simulink model "Final_Model_Building_2_AirflowAdded"  (R2022a)
settings: Solver=ode1  StartTime=0.0  StopTime=24*3600  FixedStep=10  RelTol=1e-3
values from neighbouring files (symbols this model uses):
  Aux_Threshold = 52    [Setup_Code_EWASP_VC.m]
  buildingAge = 2005    [Setup_Code_EWASP_VC.m]
  ceilingHeight = 2.4    [Setup_Code_EWASP_VC.m]
  conductiveHconnectMatrix = [ ... (first row only)    [Setup_Code_EWASP_VC.m]
  cRoofGreen = 100000    [Setup_Code_EWASP_VC.m]
  Defrost_After_Time = 30    [Setup_Code_EWASP_VC.m]
  DHWDemandProfile = occFreegainHotwaterElecTestPassiveOcc3(:,3)    [Setup_Code_EWASP_VC.m]
  Elec_Max = Elec_Max*(30/24.2)    [Setup_Code_EWASP_VC.m]
  Elec_Mid = Elec_Mid*(30/24.2)    [Setup_Code_EWASP_VC.m]
  Elec_Min = Elec_Min*(30/24.2)    [Setup_Code_EWASP_VC.m]
  ElecDemandProfile = occFreegainHotwaterElecTestPassiveOcc3(:,4)    [Setup_Code_EWASP_VC.m]
  ElecFixed = [Elec_Max(6,2) Elec_Max(6,4) Elec_Max(6,6) Elec_Max(6,7) ... (first row only)    [Setup_Code_EWASP_VC.m]
  floorOrCeilingArea = floorOrCeilingArea*1.15    [Setup_Code_EWASP_VC.m]
  forceCold = 0    [Setup_Code_EWASP_VC.m]
  freegain = occFreegainHotwaterElecTestPassiveOcc3(:,2)-max(occupancy)*25    [Setup_Code_EWASP_VC.m]
  furnitureModelOn = 1    [Setup_Code_EWASP_VC.m]
  Heat_Max = Heat_Max*(30/24.2)    [Setup_Code_EWASP_VC.m]
  Heat_Mid = Heat_Mid*(30/24.2)    [Setup_Code_EWASP_VC.m]
  Heat_Min = Heat_Min*(30/24.2)    [Setup_Code_EWASP_VC.m]
  HeatFixed = [Heat_Max(6,2) Heat_Max(6,4) Heat_Max(6,6) Heat_Max(6,7) ... (first row only)    [Setup_Code_EWASP_VC.m]
  HeatingOnProfile = repmat(HeatingOnProfile,365,1)    [Setup_Code_EWASP_VC.m]
  HEX_ReturnLowerLimit = 52.5    [Setup_Code_EWASP_VC.m]
  HEX_ReturnUpperLimit = 55    [Setup_Code_EWASP_VC.m]
  LeakMultiplier = 1+(2*(rand()-0.5)/10)    [Setup_Code_EWASP_VC.m]
  maxOcc = max(occupancyProfile)    [Setup_Code_EWASP_VC.m]
  NESW_wallArea = max(NESW_Lengths*ceilingHeight-NESW_Windows,0)    [Setup_Code_EWASP_VC.m]
  NESW_Windows = [ ... (first row only)    [Setup_Code_EWASP_VC.m]
  numRooms = roomCount    [Setup_Code_EWASP_VC.m]
  occupancy = occupancyProfile    [Setup_Code_EWASP_VC.m]
  offsetDays = 0    [Setup_Code_EWASP_VC.m]
  pumpChoice = pumpChoices(MinIndex,1)    [Setup_Code_EWASP_VC.m]
  pumpRamp = 180    [Setup_Code_EWASP_VC.m]
  ReturnLowerLimit = 37.5    [Setup_Code_EWASP_VC.m]
  ReturnUpperLimit = 40    [Setup_Code_EWASP_VC.m]
  RoofIrradiance = Flat_NS_EW_RoofIrradiance(:,1)    [Setup_Code_EWASP_VC.m]
  roofStartTemp = ones(11,1)*20    [Setup_Code_EWASP_VC.m]
  rooftype = 0    [Setup_Code_EWASP_VC.m]
  RoomDataMatrix = [zeros(1,12);ones(1,12)*wallDensity;zeros(1,12);ones(1,12)*wallU;ones(1,12)*windowU;ones(1,12)*floorU;ones(1,12)*ceilingU;zeros(1,12);windowArea, 0;floorOrCeilingArea;zeros(1,12);floorOrCeilingArea*ceilingHeight]    [Setup_Code_EWASP_VC.m]
  roomVol = roomVol*1.15    [Setup_Code_EWASP_VC.m]
  slabStartTemp = (GroundTempTimeSeries(offsetDays*1440+1,1)+thermostatSetting)/2    [Setup_Code_EWASP_VC.m]
  SlackRequest = zeros(1440,1)    [Setup_Code_EWASP_VC.m]
  SolarThermalExists = 0    [Setup_Code_EWASP_VC.m]
  SourceFixed = HeatFixed-ElecFixed    [Setup_Code_EWASP_VC.m]
  StateSeries = StateSeriesGenerator(22,7,1)    [Setup_Code_EWASP_VC.m]
  Tank_Lower_Temp = 49.5    [Setup_Code_EWASP_VC.m]
  Tank_Upper_Temp = 52    [Setup_Code_EWASP_VC.m]
  Tank_Volume_m3 = 0.15    [Setup_Code_EWASP_VC.m]
  TankHeatHour = randi([1 5])-1    [Setup_Code_EWASP_VC.m]
  upDown = [0;0;0;0;1;1;1;1;1;1;1]    [Setup_Code_EWASP_VC.m]
  wallStartTempExt = thermostatSetting*(0.266+0.00215*outdoorStartTemp+0.018*wallU+0.00113*outdoorStartTemp*wallU+0.0068*wallU^2)    [Setup_Code_EWASP_VC.m]
undefined symbols (not defined in the file or in its folder): a, ceilingU, condUDMatrix, convUDMatrix, deltaPEXPANDED_E, deltaPEXPANDED_E2, deltaPEXPANDED_N, deltaPEXPANDED_N2, deltaPEXPANDED_S, deltaPEXPANDED_S2, deltaPEXPANDED_W, deltaPEXPANDED_W2, DesiredDHWTemp, DesiredFlowTempVsInOutDeltaTemp, DiffuseHorizontal, DiscIntNeverNeededParam, DNI, dwnAndConcrete, DWORK_A_HX, DWORK_CHK_FLU, DWORK_CP_NODE, DWORK_DH, DWORK_FLUID, DWORK_HCON, DWORK_LOSS, DWORK_MDOTDOWN, DWORK_MDOTIN, DWORK_MDOTUP, DWORK_MIX, DWORK_PRESS, DWORK_QDOTIN, DWORK_RHO_NODE, DWORK_TIN, DWORK_TS_OLD, DWORK_V_NODE, ExtractRates, GroundTempTimeSeries, HCM, HCM2, HCM_closed, HCM_closed2, intermediateU, IsTop, massFlowMatrix, mechEfficiency, neighbourMatrix, numericalRoomUse, RadiatorMatrix, room2roomflowmatrix_E, room2roomflowmatrix_E2, room2roomflowmatrix_N, room2roomflowmatrix_N2, room2roomflowmatrix_S, room2roomflowmatrix_S2, room2roomflowmatrix_W, room2roomflowmatrix_W2, StateAirInEXPANDED_E, StateAirInEXPANDED_E2, StateAirInEXPANDED_N, StateAirInEXPANDED_N2 ... (+27)
libraries: simulink x6, dspsigops x4, dspmtrx3 x4, carnot x3, spsEdgeDetectorLib x2, dspstat3 x2, powerlib_meascontrol x1, simulink_extras x1
(part 16 of 27)

== system Final_Model_Building_2_AirflowAdded/Subsystem_Room3/Utility/Subsystem7 ==
  note: Q from room to ground
  In1 : Inport
  In2 : Inport  Port=2
  In3 : Inport  Port=3
  In4 : Inport  Port=4
  In5 : Inport  Port=5
  In6 : Inport  Port=6
  In7 : Inport  Port=7
  In8 : Inport  Port=8
  C per kg : Constant  Value=1000
  C per kg1 : Constant  Value=0.25
  Density : Constant  Value=2350
  Floor heat capacity total : Product  Inputs=4
  Product : Product  Inputs=3
  Product1 : Product  Inputs=3
  Product2 : Product  Inputs=*/
  QlossFromNodetoGround : Product  Inputs=3
  Sum : Sum  Inputs=+-
  Sum1 : Sum  Inputs=+-
  Sum2 : Sum
  Tchange node to ground : Product  Inputs=*/
  Thickness : Constant  Value=0.2
  deltaTNode-Ground : Sum  Inputs=+-
  doubler : Constant  Value=2
  halfUVal : Product
  "house has green roof, and the room is on the top floor" : Constant
  subtract room-concret loss from conrete-earth loss : Sum  Inputs=-+
  "switches off normal house roof loss if a green or passive roof is selected, and the room is on the top floor" : Switch  Criteria=u2 > Threshold  Threshold=0.5  SaturateOnIntegerOverflow=off  InputSameDT=off
  z : Constant  Value=0
  Out1 : Outport  VectorParamsAs1DForOutWhenUnconnected=off
  Out2 : Outport  Port=2  VectorParamsAs1DForOutWhenUnconnected=off
  wires:
  In6/1 -> Product1/3
  Sum/1 -> Product/1
  In1/1 -> Sum/1, Sum1/1
  In2/1 -> deltaTNode-Ground/2
  In4/1 -> Floor heat capacity total/1, Product1/2, Product/2, QlossFromNodetoGround/2
  Sum1/1 -> Product1/1
  "switches off normal house roof loss if a green or passive roof is selected, and the room is on the top floor"/1 -> Sum2/2
  In5/1 -> halfUVal/2
  In3/1 -> Sum1/2
  Sum2/1 -> Product2/1
  In7/1 -> Product2/2
  Product2/1 -> Out1/1
  C per kg/1 -> Floor heat capacity total/2
  Density/1 -> Floor heat capacity total/4
  Thickness/1 -> Floor heat capacity total/3
  In8/1 -> Sum/2, deltaTNode-Ground/1
  doubler/1 -> halfUVal/1
  deltaTNode-Ground/1 -> QlossFromNodetoGround/1
  halfUVal/1 -> QlossFromNodetoGround/3
  Floor heat capacity total/1 -> Tchange node to ground/2
  Product/1 -> subtract room-concret loss from conrete-earth loss/1, Sum2/1
  QlossFromNodetoGround/1 -> subtract room-concret loss from conrete-earth loss/2
  subtract room-concret loss from conrete-earth loss/1 -> Tchange node to ground/1
  Tchange node to ground/1 -> Out2/1
  C per kg1/1 -> Product/3
  Product1/1 -> "switches off normal house roof loss if a green or passive roof is selected, and the room is on the top floor"/3
  z/1 -> "switches off normal house roof loss if a green or passive roof is selected, and the room is on the top floor"/1
  "house has green roof, and the room is on the top floor"/1 -> "switches off normal house roof loss if a green or passive roof is selected, and the room is on the top floor"/2

== system Final_Model_Building_2_AirflowAdded/Subsystem_Room3/Utility/furniture ==
  In1 : Inport
  In2 : Inport  Port=2
  In3 : Inport  Port=3
  Constant3 : Constant  Value=20
  Constant4 : Constant  Value=20
  Discrete-Time Integrator : DiscreteIntegrator  InitialConditionSource=external  SampleTime=-1  ICPrevOutput=DiscIntNeverNeededParam  ICPrevScaledInput=DiscIntNeverNeededParam
  Discrete-Time Integrator1 : DiscreteIntegrator  InitialConditionSource=external  SampleTime=-1  ICPrevOutput=DiscIntNeverNeededParam  ICPrevScaledInput=DiscIntNeverNeededParam
  MATLAB Function : MATLAB Function  TreatAsAtomicUnit=on
  Plus1 : Sum
  Out1 : Outport  VectorParamsAs1DForOutWhenUnconnected=off
  wires:
  [A1] -> Discrete-Time Integrator/1
  Constant4/1 -> Discrete-Time Integrator1/2
  [B1] -> Discrete-Time Integrator1/1
  Constant3/1 -> Discrete-Time Integrator/2
  Discrete-Time Integrator/1 -> MATLAB Function/4(TemperatureWoodPlastic)
  Discrete-Time Integrator1/1 -> MATLAB Function/5(TemperatureSoft)
  MATLAB Function/2(deltaTWoodPlasticMean) -> [A1]
  MATLAB Function/4(deltaTsoftMean) -> [B1]
  MATLAB Function/3(softHeatTransfertoroom) -> Plus1/2
  MATLAB Function/1(woodPlasticHeatTransfertoroom) -> Plus1/1
  In3/1 -> MATLAB Function/3(roomTemp)
  In1/1 -> MATLAB Function/1(roomArea)
  Plus1/1 -> Out1/1
  In2/1 -> MATLAB Function/2(roomtype)

== system Final_Model_Building_2_AirflowAdded/Subsystem_Room4/Hall/Radiator w//Thermostatic Control1 ==
  In1 : Inport
  In3 : Inport  Port=2
  In2 : Inport  Port=3
  Add : Sum  Inputs=+-
  Constant : Constant  Value=Water_Volume
  Constant1 : Constant  Value=TRV_Therm_Setpoint
  Constant11 : Constant  Value=0
  Constant2 : Constant  Value=0.5
  Constant3 : Constant  Value=4180
  Constant6 : Constant  Value=40
  Constant7 : Constant  Value=40
  Discrete-Time Integrator : DiscreteIntegrator  InitialConditionSource=external  SampleTime=-1  ICPrevOutput=DiscIntNeverNeededParam  ICPrevScaledInput=DiscIntNeverNeededParam
  Discrete-Time Integrator1 : DiscreteIntegrator  InitialConditionSource=external  SampleTime=-1  ICPrevOutput=DiscIntNeverNeededParam  ICPrevScaledInput=DiscIntNeverNeededParam
  From : From
  Goto : Goto
  MATLAB Function : MATLAB Function  TreatAsAtomicUnit=on
  Product2 : Product
  Qdot2room1 : Scope
  Real-Imag to Complex : RealImagToComplex
  Saturation : Saturate  UpperLimit=1  LowerLimit=0
  Scope1 : Scope
  Sum2 : Sum
  const1 : Constant  Value=Power_Nominal
  dTnom : Constant  Value=DeltaT_Nominal
  Out3 : Outport  VectorParamsAs1DForOutWhenUnconnected=off
  Out1 : Outport  Port=2  VectorParamsAs1DForOutWhenUnconnected=off
  Out2 : Outport  Port=3  VectorParamsAs1DForOutWhenUnconnected=off
  wires:
  In1/1 -> MATLAB Function/9(Troom), Add/2
  In2/1 -> Product2/1
  Constant1/1 -> Add/1
  Add/1 -> Sum2/1
  Constant2/1 -> Sum2/2
  Sum2/1 -> Saturation/1
  Saturation/1 -> Qdot2room1/1, Product2/2
  Constant11/1 -> Real-Imag to Complex/2
  Discrete-Time Integrator/1 -> MATLAB Function/5(Tnode1)
  Real-Imag to Complex/1 -> MATLAB Function/8(nominalDeltaT)
  MATLAB Function/3(Qtoroom) -> Out3/1, Scope1/1
  Product2/1 -> MATLAB Function/3(mdotRad), Out2/1
  Constant3/1 -> MATLAB Function/2(heatCapRad)
  const1/1 -> MATLAB Function/7(nominalHeat)
  [B] -> Discrete-Time Integrator1/1
  Constant6/1 -> Discrete-Time Integrator/2
  dTnom/1 -> Real-Imag to Complex/1
  Constant7/1 -> Discrete-Time Integrator1/2
  MATLAB Function/1(deltaT1) -> Goto/1
  MATLAB Function/2(deltaT2) -> [B]
  Discrete-Time Integrator1/1 -> Out1/1, MATLAB Function/6(Tnode2)
  Constant/1 -> MATLAB Function/1(MassRad)
  In3/1 -> MATLAB Function/4(Tflow)
  From/1 -> Discrete-Time Integrator/1

== system Final_Model_Building_2_AirflowAdded/Subsystem_Room4/Hall/Subsystem1 ==
  In1 : Inport
  In2 : Inport  Port=2
  In3 : Inport  Port=3
  In4 : Inport  Port=4
  In5 : Inport  Port=5
  Add : Sum
  Constant1 : Constant  Value=TemperatureSeries
  Constant2 : Constant  Value=offsetDays
  Constant3 : Constant  Value=0.3
  Constant4 : Constant  Value=offsetDays
  Digital Clock : DigitalClock  SampleTime=10
  Digital Clock1 : DigitalClock  SampleTime=10
  MATLAB Function : MATLAB Function  TreatAsAtomicUnit=on
  MATLAB Function1 : MATLAB Function  TreatAsAtomicUnit=on
  RoomNodeNumber1 : Constant  Value=wallHeatCapacityInt
  RoomNodeNumber2 : Constant  Value=Wall_Irradiance_Angles_NEWS
  RoomNodeNumber3 : Constant  Value=DNI
  RoomNodeNumber4 : Constant  Value=DiffuseHorizontal
  RoomNodeNumber5 : Constant  Value=NESW_wallArea
  RoomNodeNumber6 : Constant  Value=NESW_wallArea
  RoomNodeNumber7 : Constant  Value=wallHeatCapacityMid
  RoomNodeNumber8 : Constant  Value=wallHeatCapacityExt
  Scope : Scope
  Scope1 : Scope
  Scope2 : Scope  NumInputPorts=3
  Scope3 : Scope
  Terminator : Terminator
  Terminator1 : Terminator
  Windspeed : Constant  Value=windSpeedSeries
  integrate deltat's with initial wall temps as initial condition : Subsystem
  sum to give HEAT LOST (i.e. positive value is a loss) : Sum  Inputs=+
  uVal_Total for wall : Constant  Value=wallU
  Out1 : Outport  VectorParamsAs1DForOutWhenUnconnected=off
  Out2 : Outport  Port=2  VectorParamsAs1DForOutWhenUnconnected=off
  Out3 : Outport  Port=3  VectorParamsAs1DForOutWhenUnconnected=off
  Out4 : Outport  Port=4  VectorParamsAs1DForOutWhenUnconnected=off
  wires:
  Constant1/1 -> MATLAB Function/9(T_AmbientSeries)
  integrate deltat's with initial wall temps as initial condition/1(Out1) -> Scope2/1, MATLAB Function/5(T_InWallNEWS)
  RoomNodeNumber2/1 -> MATLAB Function1/1(angleSeries)
  RoomNodeNumber1/1 -> MATLAB Function/2(c_InPU)
  MATLAB Function/2(deltaTmid) -> Out3/1
  In5/1 -> MATLAB Function/8(T_Room)
  MATLAB Function1/2(NEWS_Irradiance) -> Terminator1/1
  MATLAB Function/4(logRoomHeatLoss) -> sum to give HEAT LOST (i.e. positive value is a loss)/1, Scope/1
  RoomNodeNumber8/1 -> MATLAB Function/4(c_OutPU), MATLAB Function1/9(c_OutPU)
  uVal_Total for wall/1 -> MATLAB Function/1(uValWall)
  In4/1 -> integrate deltat's with initial wall temps as initial condition/3(In3)
  Digital Clock/1 -> MATLAB Function1/4(Time)
  integrate deltat's with initial wall temps as initial condition/2(Out2) -> Scope2/2, Scope1/1, MATLAB Function/6(T_MidWallNEWS)
  RoomNodeNumber7/1 -> MATLAB Function/3(c_MidPU)
  RoomNodeNumber3/1 -> MATLAB Function1/2(DNISeries)
  integrate deltat's with initial wall temps as initial condition/3(Out3) -> Scope2/3, MATLAB Function/7(T_OutWallNEWS)
  MATLAB Function/1(deltaTint) -> Out2/1
  MATLAB Function/3(deltaTout) -> Add/2
  In3/1 -> integrate deltat's with initial wall temps as initial condition/2(In2)
  Windspeed/1 -> MATLAB Function/10(windSpeedSeries)
  Constant3/1 -> MATLAB Function1/6(SurfaceAlbedo)
  RoomNodeNumber4/1 -> MATLAB Function1/3(DiffSeries)
  In1/1 -> integrate deltat's with initial wall temps as initial condition/4(In4), Scope3/1, MATLAB Function/12(roomNumber), MATLAB Function1/8(roomNumber)
  MATLAB Function1/3(deltaTexternalNEWS) -> Add/1
  RoomNodeNumber5/1 -> MATLAB Function1/7(NESW_wallArea)
  RoomNodeNumber6/1 -> MATLAB Function/11(NESW_wallArea)
  Constant4/1 -> MATLAB Function/14(offsetDays)
  Constant2/1 -> MATLAB Function1/5(offsetDays)
  Digital Clock1/1 -> MATLAB Function/13(Time)
  MATLAB Function1/1(PU_AreaIrradianceTotal) -> Terminator/1
  In2/1 -> integrate deltat's with initial wall temps as initial condition/1(In1)
  sum to give HEAT LOST (i.e. positive value is a loss)/1 -> Out4/1
  Add/1 -> Out1/1

== system Final_Model_Building_2_AirflowAdded/Subsystem_Room4/Hall/Subsystem2 ==
  In1 : Inport
  In2 : Inport  Port=2
  Constant9 : Constant  Value=-1
  Direct Lookup Table (n-D) : LookupNDDirect  NumberOfTableDimensions=1  TableIsInput=on
  Plus : Sum
  Out1 : Outport  VectorParamsAs1DForOutWhenUnconnected=off
  wires:
  Plus/1 -> Direct Lookup Table (n-D)/1
  Direct Lookup Table (n-D)/1 -> Out1/1
  Constant9/1 -> Plus/2
  In1/1 -> Plus/1
  In2/1 -> Direct Lookup Table (n-D)/2

== system Final_Model_Building_2_AirflowAdded/Subsystem_Room4/Hall/Subsystem3 ==
  In1 : Inport
  In2 : Inport  Port=2
  In3 : Inport  Port=3
  In4 : Inport  Port=4
  In5 : Inport  Port=5
  Add : Sum
  Constant1 : Constant  Value=TemperatureSeries
  Constant2 : Constant  Value=offsetDays
  Constant3 : Constant  Value=0.3
  Constant4 : Constant  Value=offsetDays
  Digital Clock : DigitalClock  SampleTime=10
  Digital Clock1 : DigitalClock  SampleTime=10
  MATLAB Function : MATLAB Function  TreatAsAtomicUnit=on
  MATLAB Function1 : MATLAB Function  TreatAsAtomicUnit=on
  RoomNodeNumber{1,3..4,7} (4 alike) : Constant  Value=cRoofGreen/3
  RoomNodeNumber2 : Constant  Value=RoofIrradiance
  RoomNodeNumber5 : Constant  Value=floorOrCeilingArea(1,4)*IsTop(1,4)
  Scope1 : Scope  NumInputPorts=3
  Scope2 : Scope  NumInputPorts=3
  Terminator : Terminator
  Windspeed : Constant  Value=windSpeedSeries
  integrate deltat's with initial wall temps as initial condition : Subsystem
  sum to give HEAT LOST (i.e. positive value is a loss) : Sum  Inputs=+
  uVal_Total for wall : Constant  Value=ceilingU
  Out1 : Outport  VectorParamsAs1DForOutWhenUnconnected=off
  Out2 : Outport  Port=2  VectorParamsAs1DForOutWhenUnconnected=off
  Out3 : Outport  Port=3  VectorParamsAs1DForOutWhenUnconnected=off
  Out4 : Outport  Port=4  VectorParamsAs1DForOutWhenUnconnected=off
  wires:
  Constant1/1 -> MATLAB Function/9(T_AmbientSeries)
  integrate deltat's with initial wall temps as initial condition/1(Out1) -> Scope2/1, MATLAB Function/5(T_InWall)
  RoomNodeNumber2/1 -> MATLAB Function1/6(RoofIrradiance)
  RoomNodeNumber4/1 -> MATLAB Function/2(c_InPU)
  MATLAB Function/2(deltaTmid) -> Scope1/2, Out3/1
  In5/1 -> MATLAB Function/8(T_Room)
  MATLAB Function/4(logRoomHeatLoss) -> sum to give HEAT LOST (i.e. positive value is a loss)/1
  RoomNodeNumber7/1 -> MATLAB Function/4(c_OutPU)
  uVal_Total for wall/1 -> MATLAB Function/1(uValWall)
  In4/1 -> integrate deltat's with initial wall temps as initial condition/3(In3)
  Digital Clock/1 -> MATLAB Function1/1(Time)
  integrate deltat's with initial wall temps as initial condition/2(Out2) -> Scope2/2, MATLAB Function/6(T_MidWall)
  RoomNodeNumber1/1 -> MATLAB Function/3(c_MidPU)
  RoomNodeNumber3/1 -> MATLAB Function1/5(c_OutRoof)
  integrate deltat's with initial wall temps as initial condition/3(Out3) -> Scope2/3, MATLAB Function/7(T_OutWall)
  MATLAB Function/1(deltaTint) -> Scope1/1, Out2/1
  MATLAB Function/3(deltaTout) -> Scope1/3, Add/2
  In3/1 -> integrate deltat's with initial wall temps as initial condition/2(In2)
  Windspeed/1 -> MATLAB Function/10(windSpeedSeries)
  Constant3/1 -> MATLAB Function1/3(SurfaceAlbedo)
  In1/1 -> integrate deltat's with initial wall temps as initial condition/4(In4), MATLAB Function/12(roomNumber)
  MATLAB Function1/2(deltaTexternal) -> Add/1
  Constant4/1 -> MATLAB Function/14(offsetDays)
  Constant2/1 -> MATLAB Function1/2(offsetDays)
  Digital Clock1/1 -> MATLAB Function/13(Time)
  MATLAB Function1/1(Tot_Irradiance) -> Terminator/1
  In2/1 -> integrate deltat's with initial wall temps as initial condition/1(In1)
  sum to give HEAT LOST (i.e. positive value is a loss)/1 -> Out4/1
  Add/1 -> Out1/1
  RoomNodeNumber5/1 -> MATLAB Function/11(ceilArea), MATLAB Function1/4(RoofArea)

== system Final_Model_Building_2_AirflowAdded/Subsystem_Room4/Hall/Subsystem4 ==
  In1 : Inport
  In2 : Inport  Port=2
  In3 : Inport  Port=3
  Constant1 : Constant  Value=[20;20;20;20]
  Constant2 : Constant  Value=offsetDays
  Constant3 : Constant  Value=90
  Constant4 : Constant  Value=[20;20;20;20]
  Digital Clock : DigitalClock  SampleTime=10
  Discrete-Time Integrator : DiscreteIntegrator  InitialConditionSource=external  SampleTime=-1  ICPrevOutput=DiscIntNeverNeededParam  ICPrevScaledInput=DiscIntNeverNeededParam
  Discrete-Time Integrator1 : DiscreteIntegrator  InitialConditionSource=external  SampleTime=-1  ICPrevOutput=DiscIntNeverNeededParam  ICPrevScaledInput=DiscIntNeverNeededParam
  Display : Display
  Display1 : Display
  Irradiance to Solar Gain1 : Subsystem
      mask Display:
      | port_label('input',1,'Incidence Angle')
      | port_label('input',2,'Tilt Angle')
      | port_label('input',3,'DNI')
      | port_label('input',4,'Diff_I')
      | port_label('output',1,'Qdot_SG')
      | port_label('output',2,'NEWS Absorbance')
      | disp('I2SG')
  MATLAB Function : MATLAB Function  TreatAsAtomicUnit=on
  MATLAB Function2 : MATLAB Function  TreatAsAtomicUnit=on
  RoomNodeNumber1 : Constant  Value=windowU
  RoomNodeNumber3 : Constant  Value=DNI
  RoomNodeNumber4 : Constant  Value=DiffuseHorizontal
  RoomNodeNumber5 : Constant  Value=NESW_Windows
  Sum of Elements : Sum  Inputs=+
  angle that DNI hits a NEWS wall/window as a function of time : Constant  Value=Wall_Irradiance_Angles_NEWS
  sum of heat GAINED by internal surfaces due to irradiance THROUGH window : Sum  Inputs=+
  Out1 : Outport  VectorParamsAs1DForOutWhenUnconnected=off
  Out2 : Outport  Port=2  VectorParamsAs1DForOutWhenUnconnected=off
  wires:
  Constant2/1 -> MATLAB Function2/5(offsetDays)
  MATLAB Function2/1(Angle_NEWS) -> Irradiance to Solar Gain1/1(In1)
  In1/1 -> MATLAB Function/8(roomNumber), MATLAB Function2/7(roomNumber)
  MATLAB Function2/2(NEWS_DNI) -> Irradiance to Solar Gain1/3(In3)
  angle that DNI hits a NEWS wall/window as a function of time/1 -> MATLAB Function2/1(angleSeries)
  sum of heat GAINED by internal surfaces due to irradiance THROUGH window/1 -> Out1/1
  Irradiance to Solar Gain1/1(Out1) -> sum of heat GAINED by internal surfaces due to irradiance THROUGH window/1
  Digital Clock/1 -> MATLAB Function2/4(Time)
  RoomNodeNumber3/1 -> MATLAB Function2/2(DNISeries)
  RoomNodeNumber4/1 -> MATLAB Function2/3(DiffSeries)
  Constant3/1 -> Irradiance to Solar Gain1/2(In2)
  RoomNodeNumber5/1 -> MATLAB Function/3(NESW_Windows), MATLAB Function2/6(NESW_Windows)
  MATLAB Function2/3(NEWS_Diff) -> Irradiance to Solar Gain1/4(In4)
  Irradiance to Solar Gain1/2(Out2) -> MATLAB Function/6(absorbedNEWS)
  In2/1 -> [Tin]
  In3/1 -> [Tout]
  [Tout] -> MATLAB Function/5(outdoorTemp)
  [Tin] -> MATLAB Function/4(roomTemp)
  RoomNodeNumber1/1 -> MATLAB Function/7(windowUval)
  [deltaT_window_In] -> Discrete-Time Integrator/1
  [deltaT_window_Out] -> Discrete-Time Integrator1/1
  Constant1/1 -> Discrete-Time Integrator/2
  Constant4/1 -> Discrete-Time Integrator1/2
  Discrete-Time Integrator/1 -> Display1/1, MATLAB Function/1(windowTempsNEWS_in)
  Discrete-Time Integrator1/1 -> MATLAB Function/2(windowTempsNEWS_out)
  MATLAB Function/1(deltaT_win_in) -> [deltaT_window_In]
  MATLAB Function/2(deltaT_win_out) -> [deltaT_window_Out]
  MATLAB Function/3(Q_to_room) -> Sum of Elements/1, Display/1
  Sum of Elements/1 -> Out2/1

== system Final_Model_Building_2_AirflowAdded/Subsystem_Room4/Hall/Subsystem6 ==
  In1 : Inport
  In2 : Inport  Port=2
  In3 : Inport  Port=3
  In4 : Inport  Port=4
  In5 : Inport  Port=5
  In6 : Inport  Port=6
  In7 : Inport  Port=7
  Product : Product  Inputs=3
  Product1 : Product  Inputs=3
  Product2 : Product  Inputs=*/
  Scope1 : Scope
  Sum : Sum  Inputs=+-
  Sum1 : Sum  Inputs=+-
  Sum2 : Sum
  "house has green roof, and the room is on the top floor" : Constant
  "switches off normal house roof loss if a green or passive roof is selected, and the room is on the top floor" : Switch  Criteria=u2 > Threshold  Threshold=0.5  SaturateOnIntegerOverflow=off  InputSameDT=off
  z : Constant  Value=0
  Out1 : Outport  VectorParamsAs1DForOutWhenUnconnected=off
  wires:
  In6/1 -> Product1/3
  Sum/1 -> Product/1
  In1/1 -> Sum1/1, Sum/1
  In2/1 -> Sum/2
  In4/1 -> Product1/2, Product/2
  Sum1/1 -> Product1/1
  Product1/1 -> Sum2/2
  In5/1 -> Product/3
  In3/1 -> Sum1/2
  Product/1 -> "switches off normal house roof loss if a green or passive roof is selected, and the room is on the top floor"/3
  Sum2/1 -> Product2/1, Scope1/1
  In7/1 -> Product2/2
  Product2/1 -> Out1/1
  z/1 -> "switches off normal house roof loss if a green or passive roof is selected, and the room is on the top floor"/1
  "house has green roof, and the room is on the top floor"/1 -> "switches off normal house roof loss if a green or passive roof is selected, and the room is on the top floor"/2
  "switches off normal house roof loss if a green or passive roof is selected, and the room is on the top floor"/1 -> Sum2/1

== system Final_Model_Building_2_AirflowAdded/Subsystem_Room4/Hall/Subsystem7 ==
  note: Q from room to ground
  In1 : Inport
  In2 : Inport  Port=2
  In3 : Inport  Port=3
  In4 : Inport  Port=4
  In5 : Inport  Port=5
  In6 : Inport  Port=6
  In7 : Inport  Port=7
  In8 : Inport  Port=8
  C per kg : Constant  Value=1000
  C per kg1 : Constant  Value=0.25
  Density : Constant  Value=2350
  Floor heat capacity total : Product  Inputs=4
  Product : Product  Inputs=3
  Product1 : Product  Inputs=3
  Product2 : Product  Inputs=*/
  QlossFromNodetoGround : Product  Inputs=3
  Scope1 : Scope
  Scope2 : Scope
  Sum : Sum  Inputs=+-
  Sum1 : Sum  Inputs=+-
  Sum2 : Sum
  Tchange node to ground : Product  Inputs=*/
  Thickness : Constant  Value=0.2
  deltaTNode-Ground : Sum  Inputs=+-
  doubler : Constant  Value=2
  halfUVal : Product
  "house has green roof, and the room is on the top floor" : Constant
  subtract room-concret loss from conrete-earth loss : Sum  Inputs=-+
  "switches off normal house roof loss if a green or passive roof is selected, and the room is on the top floor" : Switch  Criteria=u2 > Threshold  Threshold=0.5  SaturateOnIntegerOverflow=off  InputSameDT=off
  z : Constant  Value=0
  Out1 : Outport  VectorParamsAs1DForOutWhenUnconnected=off
  Out2 : Outport  Port=2  VectorParamsAs1DForOutWhenUnconnected=off
  wires:
  In6/1 -> Product1/3
  Sum/1 -> Product/1
  In1/1 -> Sum/1, Sum1/1
  In2/1 -> deltaTNode-Ground/2
  In4/1 -> Floor heat capacity total/1, Product1/2, Product/2, QlossFromNodetoGround/2
  Sum1/1 -> Product1/1
  "switches off normal house roof loss if a green or passive roof is selected, and the room is on the top floor"/1 -> Scope2/1, Sum2/2
  In5/1 -> halfUVal/2
  In3/1 -> Sum1/2
  Sum2/1 -> Product2/1
  In7/1 -> Product2/2
  Product2/1 -> Out1/1
  C per kg/1 -> Floor heat capacity total/2
  Density/1 -> Floor heat capacity total/4
  Thickness/1 -> Floor heat capacity total/3
  In8/1 -> Sum/2, deltaTNode-Ground/1
  doubler/1 -> halfUVal/1
  deltaTNode-Ground/1 -> QlossFromNodetoGround/1
  halfUVal/1 -> QlossFromNodetoGround/3
  Floor heat capacity total/1 -> Tchange node to ground/2
  Product/1 -> Scope1/1, subtract room-concret loss from conrete-earth loss/1, Sum2/1
  QlossFromNodetoGround/1 -> subtract room-concret loss from conrete-earth loss/2
  subtract room-concret loss from conrete-earth loss/1 -> Tchange node to ground/1
  Tchange node to ground/1 -> Out2/1
  C per kg1/1 -> Product/3
  Product1/1 -> "switches off normal house roof loss if a green or passive roof is selected, and the room is on the top floor"/3
  z/1 -> "switches off normal house roof loss if a green or passive roof is selected, and the room is on the top floor"/1
  "house has green roof, and the room is on the top floor"/1 -> "switches off normal house roof loss if a green or passive roof is selected, and the room is on the top floor"/2

== system Final_Model_Building_2_AirflowAdded/Subsystem_Room4/Hall/furniture ==
  In1 : Inport
  In2 : Inport  Port=2
  In3 : Inport  Port=3
  Constant3 : Constant  Value=20
  Constant4 : Constant  Value=20
  Discrete-Time Integrator : DiscreteIntegrator  InitialConditionSource=external  SampleTime=-1  ICPrevOutput=DiscIntNeverNeededParam  ICPrevScaledInput=DiscIntNeverNeededParam
  Discrete-Time Integrator1 : DiscreteIntegrator  InitialConditionSource=external  SampleTime=-1  ICPrevOutput=DiscIntNeverNeededParam  ICPrevScaledInput=DiscIntNeverNeededParam
  MATLAB Function : MATLAB Function  TreatAsAtomicUnit=on
  Plus1 : Sum
  Out1 : Outport  VectorParamsAs1DForOutWhenUnconnected=off
  wires:
  [A1] -> Discrete-Time Integrator/1
  Constant4/1 -> Discrete-Time Integrator1/2
  [B1] -> Discrete-Time Integrator1/1
  Constant3/1 -> Discrete-Time Integrator/2
  Discrete-Time Integrator/1 -> MATLAB Function/4(TemperatureWoodPlastic)
  Discrete-Time Integrator1/1 -> MATLAB Function/5(TemperatureSoft)
  MATLAB Function/2(deltaTWoodPlasticMean) -> [A1]
  MATLAB Function/4(deltaTsoftMean) -> [B1]
  MATLAB Function/3(softHeatTransfertoroom) -> Plus1/2
  MATLAB Function/1(woodPlasticHeatTransfertoroom) -> Plus1/1
  In3/1 -> MATLAB Function/3(roomTemp)
  In1/1 -> MATLAB Function/1(roomArea)
  Plus1/1 -> Out1/1
  In2/1 -> MATLAB Function/2(roomtype)

== system Final_Model_Building_2_AirflowAdded/Subsystem_Room5/Landing/Radiator w//Thermostatic Control2 ==
  In1 : Inport
  In3 : Inport  Port=2
  In2 : Inport  Port=3
  Add : Sum  Inputs=+-
  Constant : Constant  Value=Water_Volume
  Constant1 : Constant  Value=TRV_Therm_Setpoint
  Constant11 : Constant  Value=0
  Constant2 : Constant  Value=0.5
  Constant3 : Constant  Value=4180
  Constant6 : Constant  Value=40
  Constant7 : Constant  Value=40
  Discrete-Time Integrator : DiscreteIntegrator  InitialConditionSource=external  SampleTime=-1  ICPrevOutput=DiscIntNeverNeededParam  ICPrevScaledInput=DiscIntNeverNeededParam
  Discrete-Time Integrator1 : DiscreteIntegrator  InitialConditionSource=external  SampleTime=-1  ICPrevOutput=DiscIntNeverNeededParam  ICPrevScaledInput=DiscIntNeverNeededParam
  From : From
  Goto : Goto
  MATLAB Function : MATLAB Function  TreatAsAtomicUnit=on
  Product2 : Product
  Qdot2room1 : Scope
  Real-Imag to Complex : RealImagToComplex
  Saturation : Saturate  UpperLimit=1  LowerLimit=0
  Scope1 : Scope
  Sum2 : Sum
  const1 : Constant  Value=Power_Nominal
  dTnom : Constant  Value=DeltaT_Nominal
  Out3 : Outport  VectorParamsAs1DForOutWhenUnconnected=off
  Out1 : Outport  Port=2  VectorParamsAs1DForOutWhenUnconnected=off
  Out2 : Outport  Port=3  VectorParamsAs1DForOutWhenUnconnected=off
  wires:
  In1/1 -> MATLAB Function/9(Troom), Add/2
  In2/1 -> Product2/1
  Constant1/1 -> Add/1
  Add/1 -> Sum2/1
  Constant2/1 -> Sum2/2
  Sum2/1 -> Saturation/1
  Saturation/1 -> Qdot2room1/1, Product2/2
  Constant11/1 -> Real-Imag to Complex/2
  Discrete-Time Integrator/1 -> MATLAB Function/5(Tnode1)
  Real-Imag to Complex/1 -> MATLAB Function/8(nominalDeltaT)
  MATLAB Function/3(Qtoroom) -> Out3/1, Scope1/1
  Product2/1 -> MATLAB Function/3(mdotRad), Out2/1
  Constant3/1 -> MATLAB Function/2(heatCapRad)
  const1/1 -> MATLAB Function/7(nominalHeat)
  [B] -> Discrete-Time Integrator1/1
  Constant6/1 -> Discrete-Time Integrator/2
  dTnom/1 -> Real-Imag to Complex/1
  Constant7/1 -> Discrete-Time Integrator1/2
  MATLAB Function/1(deltaT1) -> Goto/1
  MATLAB Function/2(deltaT2) -> [B]
  Discrete-Time Integrator1/1 -> Out1/1, MATLAB Function/6(Tnode2)
  Constant/1 -> MATLAB Function/1(MassRad)
  In3/1 -> MATLAB Function/4(Tflow)
  From/1 -> Discrete-Time Integrator/1

== system Final_Model_Building_2_AirflowAdded/Subsystem_Room5/Landing/Subsystem ==
  In1 : Inport
  In2 : Inport  Port=2
  In3 : Inport  Port=3
  In4 : Inport  Port=4
  In5 : Inport  Port=5
  In6 : Inport  Port=6
  In7 : Inport  Port=7
  Product : Product  Inputs=3
  Product1 : Product  Inputs=3
  Product2 : Product  Inputs=*/
  Sum : Sum  Inputs=+-
  Sum1 : Sum  Inputs=+-
  Sum2 : Sum
  Out1 : Outport  VectorParamsAs1DForOutWhenUnconnected=off
  wires:
  In6/1 -> Product1/3
  Sum/1 -> Product/1
  In1/1 -> Sum1/1, Sum/1
  In2/1 -> Sum/2
  In4/1 -> Product1/2, Product/2
  Sum1/1 -> Product1/1
  Product1/1 -> Sum2/2
  In5/1 -> Product/3
  In3/1 -> Sum1/2
  Product/1 -> Sum2/1
  Sum2/1 -> Product2/1
  In7/1 -> Product2/2
  Product2/1 -> Out1/1

== system Final_Model_Building_2_AirflowAdded/Subsystem_Room5/Landing/Subsystem1 ==
  In1 : Inport
  In2 : Inport  Port=2
  In3 : Inport  Port=3
  Constant1 : Constant  Value=[20;20;20;20]
  Constant2 : Constant  Value=offsetDays
  Constant3 : Constant  Value=90
  Constant4 : Constant  Value=[20;20;20;20]
  Digital Clock : DigitalClock  SampleTime=10
  Discrete-Time Integrator : DiscreteIntegrator  InitialConditionSource=external  SampleTime=-1  ICPrevOutput=DiscIntNeverNeededParam  ICPrevScaledInput=DiscIntNeverNeededParam
  Discrete-Time Integrator1 : DiscreteIntegrator  InitialConditionSource=external  SampleTime=-1  ICPrevOutput=DiscIntNeverNeededParam  ICPrevScaledInput=DiscIntNeverNeededParam
  Display : Display
  Display1 : Display
  Irradiance to Solar Gain1 : Subsystem
      mask Display:
      | port_label('input',1,'Incidence Angle')
      | port_label('input',2,'Tilt Angle')
      | port_label('input',3,'DNI')
      | port_label('input',4,'Diff_I')
      | port_label('output',1,'Qdot_SG')
      | port_label('output',2,'NEWS Absorbance')
      | disp('I2SG')
  MATLAB Function : MATLAB Function  TreatAsAtomicUnit=on
  MATLAB Function2 : MATLAB Function  TreatAsAtomicUnit=on
  RoomNodeNumber1 : Constant  Value=windowU
  RoomNodeNumber3 : Constant  Value=DNI
  RoomNodeNumber4 : Constant  Value=DiffuseHorizontal
  RoomNodeNumber5 : Constant  Value=NESW_Windows
  Sum of Elements : Sum  Inputs=+
  angle that DNI hits a NEWS wall/window as a function of time : Constant  Value=Wall_Irradiance_Angles_NEWS
  sum of heat GAINED by internal surfaces due to irradiance THROUGH window : Sum  Inputs=+
  Out1 : Outport  VectorParamsAs1DForOutWhenUnconnected=off
  Out2 : Outport  Port=2  VectorParamsAs1DForOutWhenUnconnected=off
  wires:
  Constant2/1 -> MATLAB Function2/5(offsetDays)
  MATLAB Function2/1(Angle_NEWS) -> Irradiance to Solar Gain1/1(In1)
  In1/1 -> MATLAB Function/8(roomNumber), MATLAB Function2/7(roomNumber)
  MATLAB Function2/2(NEWS_DNI) -> Irradiance to Solar Gain1/3(In3)
  angle that DNI hits a NEWS wall/window as a function of time/1 -> MATLAB Function2/1(angleSeries)
  sum of heat GAINED by internal surfaces due to irradiance THROUGH window/1 -> Out1/1
  Irradiance to Solar Gain1/1(Out1) -> sum of heat GAINED by internal surfaces due to irradiance THROUGH window/1
  Digital Clock/1 -> MATLAB Function2/4(Time)
  RoomNodeNumber3/1 -> MATLAB Function2/2(DNISeries)
  RoomNodeNumber4/1 -> MATLAB Function2/3(DiffSeries)
  Constant3/1 -> Irradiance to Solar Gain1/2(In2)
  RoomNodeNumber5/1 -> MATLAB Function/3(NESW_Windows), MATLAB Function2/6(NESW_Windows)
  MATLAB Function2/3(NEWS_Diff) -> Irradiance to Solar Gain1/4(In4)
  Irradiance to Solar Gain1/2(Out2) -> MATLAB Function/6(absorbedNEWS)
  In2/1 -> [Tin]
  In3/1 -> [Tout]
  [Tout] -> MATLAB Function/5(outdoorTemp)
  [Tin] -> MATLAB Function/4(roomTemp)
  RoomNodeNumber1/1 -> MATLAB Function/7(windowUval)
  [deltaT_window_In] -> Discrete-Time Integrator/1
  [deltaT_window_Out] -> Discrete-Time Integrator1/1
  Constant1/1 -> Discrete-Time Integrator/2
  Constant4/1 -> Discrete-Time Integrator1/2
  Discrete-Time Integrator/1 -> Display1/1, MATLAB Function/1(windowTempsNEWS_in)
  Discrete-Time Integrator1/1 -> MATLAB Function/2(windowTempsNEWS_out)
  MATLAB Function/1(deltaT_win_in) -> [deltaT_window_In]
  MATLAB Function/2(deltaT_win_out) -> [deltaT_window_Out]
  MATLAB Function/3(Q_to_room) -> Sum of Elements/1, Display/1
  Sum of Elements/1 -> Out2/1

== system Final_Model_Building_2_AirflowAdded/Subsystem_Room5/Landing/Subsystem2 ==
  In1 : Inport
  In2 : Inport  Port=2
  In3 : Inport  Port=3
  In4 : Inport  Port=4
  In5 : Inport  Port=5
  Add : Sum
  Constant1 : Constant  Value=TemperatureSeries
  Constant2 : Constant  Value=offsetDays
  Constant3 : Constant  Value=0.3
  Constant4 : Constant  Value=offsetDays
  Digital Clock : DigitalClock  SampleTime=10
  Digital Clock1 : DigitalClock  SampleTime=10
  MATLAB Function : MATLAB Function  TreatAsAtomicUnit=on
  MATLAB Function1 : MATLAB Function  TreatAsAtomicUnit=on
  RoomNodeNumber1 : Constant  Value=wallHeatCapacityInt
  RoomNodeNumber2 : Constant  Value=Wall_Irradiance_Angles_NEWS
  RoomNodeNumber3 : Constant  Value=DNI
  RoomNodeNumber4 : Constant  Value=DiffuseHorizontal
  RoomNodeNumber5 : Constant  Value=NESW_wallArea
  RoomNodeNumber6 : Constant  Value=NESW_wallArea
  RoomNodeNumber7 : Constant  Value=wallHeatCapacityMid
  RoomNodeNumber8 : Constant  Value=wallHeatCapacityExt
  Scope : Scope
  Scope1 : Scope
  Scope2 : Scope  NumInputPorts=3
  Scope3 : Scope
  Terminator : Terminator
  Terminator1 : Terminator
  Windspeed : Constant  Value=windSpeedSeries
  integrate deltat's with initial wall temps as initial condition : Subsystem
  sum to give HEAT LOST (i.e. positive value is a loss) : Sum  Inputs=+
  uVal_Total for wall : Constant  Value=wallU
  Out1 : Outport  VectorParamsAs1DForOutWhenUnconnected=off
  Out2 : Outport  Port=2  VectorParamsAs1DForOutWhenUnconnected=off
  Out3 : Outport  Port=3  VectorParamsAs1DForOutWhenUnconnected=off
  Out4 : Outport  Port=4  VectorParamsAs1DForOutWhenUnconnected=off
  wires:
  Constant1/1 -> MATLAB Function/9(T_AmbientSeries)
  integrate deltat's with initial wall temps as initial condition/1(Out1) -> Scope2/1, MATLAB Function/5(T_InWallNEWS)
  RoomNodeNumber2/1 -> MATLAB Function1/1(angleSeries)
  RoomNodeNumber1/1 -> MATLAB Function/2(c_InPU)
  MATLAB Function/2(deltaTmid) -> Out3/1
  In5/1 -> MATLAB Function/8(T_Room)
  MATLAB Function1/2(NEWS_Irradiance) -> Terminator1/1
  MATLAB Function/4(logRoomHeatLoss) -> sum to give HEAT LOST (i.e. positive value is a loss)/1, Scope/1
  RoomNodeNumber8/1 -> MATLAB Function/4(c_OutPU), MATLAB Function1/9(c_OutPU)
  uVal_Total for wall/1 -> MATLAB Function/1(uValWall)
  In4/1 -> integrate deltat's with initial wall temps as initial condition/3(In3)
  Digital Clock/1 -> MATLAB Function1/4(Time)
  integrate deltat's with initial wall temps as initial condition/2(Out2) -> Scope2/2, Scope1/1, MATLAB Function/6(T_MidWallNEWS)
  RoomNodeNumber7/1 -> MATLAB Function/3(c_MidPU)
  RoomNodeNumber3/1 -> MATLAB Function1/2(DNISeries)
  integrate deltat's with initial wall temps as initial condition/3(Out3) -> Scope2/3, MATLAB Function/7(T_OutWallNEWS)
  MATLAB Function/1(deltaTint) -> Out2/1
  MATLAB Function/3(deltaTout) -> Add/2
  In3/1 -> integrate deltat's with initial wall temps as initial condition/2(In2)
  Windspeed/1 -> MATLAB Function/10(windSpeedSeries)
  Constant3/1 -> MATLAB Function1/6(SurfaceAlbedo)
  RoomNodeNumber4/1 -> MATLAB Function1/3(DiffSeries)
  In1/1 -> integrate deltat's with initial wall temps as initial condition/4(In4), Scope3/1, MATLAB Function/12(roomNumber), MATLAB Function1/8(roomNumber)
  MATLAB Function1/3(deltaTexternalNEWS) -> Add/1
  RoomNodeNumber5/1 -> MATLAB Function1/7(NESW_wallArea)
  RoomNodeNumber6/1 -> MATLAB Function/11(NESW_wallArea)
  Constant4/1 -> MATLAB Function/14(offsetDays)
  Constant2/1 -> MATLAB Function1/5(offsetDays)
  Digital Clock1/1 -> MATLAB Function/13(Time)
  MATLAB Function1/1(PU_AreaIrradianceTotal) -> Terminator/1
  In2/1 -> integrate deltat's with initial wall temps as initial condition/1(In1)
  sum to give HEAT LOST (i.e. positive value is a loss)/1 -> Out4/1
  Add/1 -> Out1/1

== system Final_Model_Building_2_AirflowAdded/Subsystem_Room5/Landing/Subsystem3 ==
  In1 : Inport
  In2 : Inport  Port=2
  In3 : Inport  Port=3
  In4 : Inport  Port=4
  In5 : Inport  Port=5
  Add : Sum
  Constant1 : Constant  Value=TemperatureSeries
  Constant2 : Constant  Value=offsetDays
  Constant3 : Constant  Value=0.3
  Constant4 : Constant  Value=offsetDays
  Digital Clock : DigitalClock  SampleTime=10
  Digital Clock1 : DigitalClock  SampleTime=10
  MATLAB Function : MATLAB Function  TreatAsAtomicUnit=on
  MATLAB Function1 : MATLAB Function  TreatAsAtomicUnit=on
  RoomNodeNumber{1,3..4,7} (4 alike) : Constant  Value=cRoofGreen/3
  RoomNodeNumber2 : Constant  Value=RoofIrradiance
  RoomNodeNumber5 : Constant  Value=floorOrCeilingArea(1,5)*IsTop(1,5)
  Scope1 : Scope  NumInputPorts=3
  Scope2 : Scope  NumInputPorts=3
  Terminator : Terminator
  Windspeed : Constant  Value=windSpeedSeries
  integrate deltat's with initial wall temps as initial condition : Subsystem
  sum to give HEAT LOST (i.e. positive value is a loss) : Sum  Inputs=+
  uVal_Total for wall : Constant  Value=ceilingU
  Out1 : Outport  VectorParamsAs1DForOutWhenUnconnected=off
  Out2 : Outport  Port=2  VectorParamsAs1DForOutWhenUnconnected=off
  Out3 : Outport  Port=3  VectorParamsAs1DForOutWhenUnconnected=off
  Out4 : Outport  Port=4  VectorParamsAs1DForOutWhenUnconnected=off
  wires:
  Constant1/1 -> MATLAB Function/9(T_AmbientSeries)
  integrate deltat's with initial wall temps as initial condition/1(Out1) -> Scope2/1, MATLAB Function/5(T_InWall)
  RoomNodeNumber2/1 -> MATLAB Function1/6(RoofIrradiance)
  RoomNodeNumber4/1 -> MATLAB Function/2(c_InPU)
  MATLAB Function/2(deltaTmid) -> Scope1/2, Out3/1
  In5/1 -> MATLAB Function/8(T_Room)
  MATLAB Function/4(logRoomHeatLoss) -> sum to give HEAT LOST (i.e. positive value is a loss)/1
  RoomNodeNumber7/1 -> MATLAB Function/4(c_OutPU)
  uVal_Total for wall/1 -> MATLAB Function/1(uValWall)
  In4/1 -> integrate deltat's with initial wall temps as initial condition/3(In3)
  Digital Clock/1 -> MATLAB Function1/1(Time)
  integrate deltat's with initial wall temps as initial condition/2(Out2) -> Scope2/2, MATLAB Function/6(T_MidWall)
  RoomNodeNumber1/1 -> MATLAB Function/3(c_MidPU)
  RoomNodeNumber3/1 -> MATLAB Function1/5(c_OutRoof)
  integrate deltat's with initial wall temps as initial condition/3(Out3) -> Scope2/3, MATLAB Function/7(T_OutWall)
  MATLAB Function/1(deltaTint) -> Scope1/1, Out2/1
  MATLAB Function/3(deltaTout) -> Scope1/3, Add/2
  In3/1 -> integrate deltat's with initial wall temps as initial condition/2(In2)
  Windspeed/1 -> MATLAB Function/10(windSpeedSeries)
  Constant3/1 -> MATLAB Function1/3(SurfaceAlbedo)
  In1/1 -> integrate deltat's with initial wall temps as initial condition/4(In4), MATLAB Function/12(roomNumber)
  MATLAB Function1/2(deltaTexternal) -> Add/1
  Constant4/1 -> MATLAB Function/14(offsetDays)
  Constant2/1 -> MATLAB Function1/2(offsetDays)
  Digital Clock1/1 -> MATLAB Function/13(Time)
  MATLAB Function1/1(Tot_Irradiance) -> Terminator/1
  In2/1 -> integrate deltat's with initial wall temps as initial condition/1(In1)
  sum to give HEAT LOST (i.e. positive value is a loss)/1 -> Out4/1
  Add/1 -> Out1/1
  RoomNodeNumber5/1 -> MATLAB Function/11(ceilArea), MATLAB Function1/4(RoofArea)

== system Final_Model_Building_2_AirflowAdded/Subsystem_Room5/Landing/Subsystem4 ==
  In1 : Inport
  In2 : Inport  Port=2
  Constant9 : Constant  Value=-1
  Direct Lookup Table (n-D) : LookupNDDirect  NumberOfTableDimensions=1  TableIsInput=on
  Plus : Sum
  Out1 : Outport  VectorParamsAs1DForOutWhenUnconnected=off
  wires:
  Plus/1 -> Direct Lookup Table (n-D)/1
  Direct Lookup Table (n-D)/1 -> Out1/1
  Constant9/1 -> Plus/2
  In1/1 -> Plus/1
  In2/1 -> Direct Lookup Table (n-D)/2

== system Final_Model_Building_2_AirflowAdded/Subsystem_Room5/Landing/Subsystem6 ==
  In1 : Inport
  In2 : Inport  Port=2
  In3 : Inport  Port=3
  In4 : Inport  Port=4
  In5 : Inport  Port=5
  In6 : Inport  Port=6
  In7 : Inport  Port=7
  Product : Product  Inputs=3
  Product1 : Product  Inputs=3
  Product2 : Product  Inputs=*/
  Scope1 : Scope
  Sum : Sum  Inputs=+-
  Sum1 : Sum  Inputs=+-
  Sum2 : Sum
  "house has green roof, and the room is on the top floor" : Constant
  "switches off normal house roof loss if a green or passive roof is selected, and the room is on the top floor" : Switch  Criteria=u2 > Threshold  Threshold=0.5  SaturateOnIntegerOverflow=off  InputSameDT=off
  z : Constant  Value=0
  Out1 : Outport  VectorParamsAs1DForOutWhenUnconnected=off
  wires:
  In6/1 -> Product1/3
  Sum/1 -> Product/1
  In1/1 -> Sum1/1, Sum/1
  In2/1 -> Sum/2
  In4/1 -> Product1/2, Product/2
  Sum1/1 -> Product1/1
  Product1/1 -> Sum2/2
  In5/1 -> Product/3
  In3/1 -> Sum1/2
  Product/1 -> "switches off normal house roof loss if a green or passive roof is selected, and the room is on the top floor"/3
  Sum2/1 -> Product2/1, Scope1/1
  In7/1 -> Product2/2
  Product2/1 -> Out1/1
  z/1 -> "switches off normal house roof loss if a green or passive roof is selected, and the room is on the top floor"/1
  "house has green roof, and the room is on the top floor"/1 -> "switches off normal house roof loss if a green or passive roof is selected, and the room is on the top floor"/2
  "switches off normal house roof loss if a green or passive roof is selected, and the room is on the top floor"/1 -> Sum2/1

== system Final_Model_Building_2_AirflowAdded/Subsystem_Room5/Landing/Subsystem7 ==
  note: Q from room to ground
  In1 : Inport
  In2 : Inport  Port=2
  In3 : Inport  Port=3
  In4 : Inport  Port=4
  In5 : Inport  Port=5
  In6 : Inport  Port=6
  In7 : Inport  Port=7
  In8 : Inport  Port=8
  C per kg : Constant  Value=1000
  C per kg1 : Constant  Value=0.25
  Density : Constant  Value=2350
  Floor heat capacity total : Product  Inputs=4
  Product : Product  Inputs=3
  Product1 : Product  Inputs=3
  Product2 : Product  Inputs=*/
  QlossFromNodetoGround : Product  Inputs=3
  Scope1 : Scope
  Scope2 : Scope
  Sum : Sum  Inputs=+-
  Sum1 : Sum  Inputs=+-
  Sum2 : Sum
  Tchange node to ground : Product  Inputs=*/
  Thickness : Constant  Value=0.2
  deltaTNode-Ground : Sum  Inputs=+-
  doubler : Constant  Value=2
  halfUVal : Product
  "house has green roof, and the room is on the top floor" : Constant
  subtract room-concret loss from conrete-earth loss : Sum  Inputs=-+
  "switches off normal house roof loss if a green or passive roof is selected, and the room is on the top floor" : Switch  Criteria=u2 > Threshold  Threshold=0.5  SaturateOnIntegerOverflow=off  InputSameDT=off
  z : Constant  Value=0
  Out1 : Outport  VectorParamsAs1DForOutWhenUnconnected=off
  Out2 : Outport  Port=2  VectorParamsAs1DForOutWhenUnconnected=off
  wires:
  In6/1 -> Product1/3
  Sum/1 -> Product/1
  In1/1 -> Sum/1, Sum1/1
  In2/1 -> deltaTNode-Ground/2
  In4/1 -> Floor heat capacity total/1, Product1/2, Product/2, QlossFromNodetoGround/2
  Sum1/1 -> Product1/1
  "switches off normal house roof loss if a green or passive roof is selected, and the room is on the top floor"/1 -> Scope2/1, Sum2/2
  In5/1 -> halfUVal/2
  In3/1 -> Sum1/2
  Sum2/1 -> Product2/1
  In7/1 -> Product2/2
  Product2/1 -> Out1/1
  C per kg/1 -> Floor heat capacity total/2
  Density/1 -> Floor heat capacity total/4
  Thickness/1 -> Floor heat capacity total/3
  In8/1 -> Sum/2, deltaTNode-Ground/1
  doubler/1 -> halfUVal/1
  deltaTNode-Ground/1 -> QlossFromNodetoGround/1
  halfUVal/1 -> QlossFromNodetoGround/3
  Floor heat capacity total/1 -> Tchange node to ground/2
  Product/1 -> Scope1/1, subtract room-concret loss from conrete-earth loss/1, Sum2/1
  QlossFromNodetoGround/1 -> subtract room-concret loss from conrete-earth loss/2
  subtract room-concret loss from conrete-earth loss/1 -> Tchange node to ground/1
  Tchange node to ground/1 -> Out2/1
  C per kg1/1 -> Product/3
  Product1/1 -> "switches off normal house roof loss if a green or passive roof is selected, and the room is on the top floor"/3
  z/1 -> "switches off normal house roof loss if a green or passive roof is selected, and the room is on the top floor"/1
  "house has green roof, and the room is on the top floor"/1 -> "switches off normal house roof loss if a green or passive roof is selected, and the room is on the top floor"/2

== system Final_Model_Building_2_AirflowAdded/Subsystem_Room5/Landing/furniture ==
  In1 : Inport
  In2 : Inport  Port=2
  In3 : Inport  Port=3
  Constant3 : Constant  Value=20
  Constant4 : Constant  Value=20
  Discrete-Time Integrator : DiscreteIntegrator  InitialConditionSource=external  SampleTime=-1  ICPrevOutput=DiscIntNeverNeededParam  ICPrevScaledInput=DiscIntNeverNeededParam
  Discrete-Time Integrator1 : DiscreteIntegrator  InitialConditionSource=external  SampleTime=-1  ICPrevOutput=DiscIntNeverNeededParam  ICPrevScaledInput=DiscIntNeverNeededParam
  MATLAB Function : MATLAB Function  TreatAsAtomicUnit=on
  Plus1 : Sum
  Out1 : Outport  VectorParamsAs1DForOutWhenUnconnected=off
  wires:
  [A1] -> Discrete-Time Integrator/1
  Constant4/1 -> Discrete-Time Integrator1/2
  [B1] -> Discrete-Time Integrator1/1
  Constant3/1 -> Discrete-Time Integrator/2
  Discrete-Time Integrator/1 -> MATLAB Function/4(TemperatureWoodPlastic)
  Discrete-Time Integrator1/1 -> MATLAB Function/5(TemperatureSoft)
  MATLAB Function/2(deltaTWoodPlasticMean) -> [A1]
  MATLAB Function/4(deltaTsoftMean) -> [B1]
  MATLAB Function/3(softHeatTransfertoroom) -> Plus1/2
  MATLAB Function/1(woodPlasticHeatTransfertoroom) -> Plus1/1
  In3/1 -> MATLAB Function/3(roomTemp)
  In1/1 -> MATLAB Function/1(roomArea)
  Plus1/1 -> Out1/1
  In2/1 -> MATLAB Function/2(roomtype)
